simulink model "test4"  (R2021a)
settings: Solver=VariableStepAuto  StartTime=0.0  StopTime=20  RelTol=1e-1
undefined symbols (not defined in the file): B_EMB, C1, C_EMB, D_EMB, f, i_EMB, JL, JM, Jm_EMB, K1, N_EMB, rb_EMB, s_EMB, sigbuilder_block, Tc_EMB, Ts_EMB, ub_EMB
libraries: powerlib_extras x9, spsDCVoltageSourceLib x5, spsPermanentMagnetSynchronousMachineLib x5, spsUniversalBridgeLib x5, spspowerguiLib x5, spsVoltageMeasurementLib x4, pid_lib x4, simulink x3, dsparch4 x2, instrumentlib x2, Solver_SF x1
(part 2 of 3)

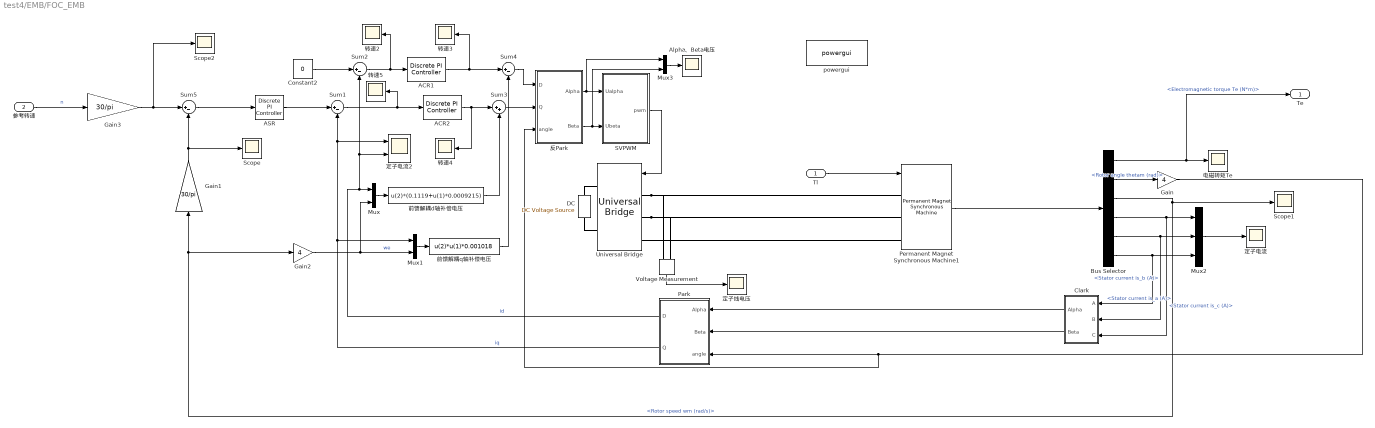
== system test4/EMB/FOC_EMB ==
  Tl : Inport
  参考转速 : Inport  Port=2
  ACR1 : powerlib_extras/Discrete  Control Blocks/Discrete PI Controller  Kp=4  Ki=80  Par_Limits=[560*0.9*sqrt(1/3) -560*0.9*sqrt(1/3)]  Init=0  Ts=1e-6
  ACR2 : powerlib_extras/Discrete  Control Blocks/Discrete PI Controller  Kp=4  Ki=80  Par_Limits=[560*0.9*sqrt(1/3) -560*0.9*sqrt(1/3)]  Init=0  Ts=1e-6
  ASR : powerlib_extras/Discrete  Control Blocks/Discrete PI Controller  Kp=5  Ki=200  Par_Limits=[65 -65]  Init=0  Ts=1e-6
  Alpha、Beta电压 : Scope
  Bus Selector : BusSelector  OutputSignals=Electromagnetic torque Te (N*m),Rotor angle thetam (rad),Rotor speed wm (rad/s),Stator current is_c (A),Stator current is_b (A),Stator current is_a (A)
  Clark : Subsystem
  Constant2 : Constant  Value=0
  DC : spsDCVoltageSourceLib/DC Voltage Source  Amplitude=560  Measurements=None
  Gain : Gain  Gain=4
  Gain1 : Gain  Gain=30/pi
  Gain2 : Gain  Gain=4
  Gain3 : Gain  Gain=30/pi
  Mux : Mux  Inputs=2
  Mux1 : Mux  Inputs=2
  Mux2 : Mux  Inputs=3
  Mux3 : Mux  Inputs=2
  Park : Subsystem
  Permanent Magnet Synchronous Machine1 : spsPermanentMagnetSynchronousMachineLib/Permanent Magnet Synchronous Machine  NbPhases=3  FluxDistribution=Sinusoidal  RotorType=Salient-pole  MechanicalLoad=Torque Tm  PresetModel=No  ShowDetailedParameters=on  MeasurementBus=off  Resistance=0.11  Inductance=8.5e-3  dqInductances=[0.0009215 0.001018]  La=0.000835  MachineConstant=Flux linkage established by magnets (V.s)  Flux=0.1119  VoltageCst=81.1857  TorqueCst=0.6714  Flat=120  Mechanical=[0.04 0.0002024 4 0]  PolePairs=4  InitialConditions=[0,0, 0,0]  InitialConditions5ph=[0 0 0 0 0 0]  RefAngle=Aligned with phase A axis (original Park)  IterativeDiscreteModel=Trapezoidal non iterative  TsBlock=-1  TsPowergui=0
  SVPWM : Subsystem
  Scope : Scope
  Scope1 : Scope
  Scope2 : Scope
  Sum{1..2,4..5} (4 alike) : Sum  Inputs=|+-
  Sum3 : Sum  Inputs=|++
  Universal Bridge : spsUniversalBridgeLib/Universal Bridge  Arms=3  SnubberResistance=1e5  SnubberCapacitance=inf  Device=IGBT / Diodes  Ron=1e-3  Lon=0  ForwardVoltages="[  0  0  ]"  ForwardVoltage=0  GTOparameters=[ 10e-6 , 20e-6 ]  IGBTparameters=[ 1e-6 , 2e-6 ]  Measurements=None  Measurements_2=None  converterType=Rectifier
  Voltage Measurement : spsVoltageMeasurementLib/Voltage Measurement  PhasorSimulation=off  OutputType=Complex  PSBequivalent=0
  powergui : spspowerguiLib/powergui  Priority=1  SimulationMode=Discrete  SampleTime=1e-6  frequency=60  Iterations=50  frequencyindice=0  Pbase=100e6  ErrMax=1e-4  UnitsV=kV  UnitsW=MW  buscounter=0  FunctionMessages=off  echomessages=off  EnableUseOfTLC=off  CurrentSourceSwitches=off  DisableSnubberDevices=off  DisableRonSwitches=off  DisableVfSwitches=off  DisplayEquations=off  AutomaticDiscreteSolvers=off  SolverType=Tustin  Interpol=off  ExternalGateDelay=off  methode=off  Ts=0  x0status=blocks  SPID=off  SwTol=0  HookPort=off  NonlinearTolerance=1e-4  nMaxIteration=100  ContinueOnMaxIteration=off  RestoreLinks=warning  ResistiveCurrentMeasurement=off  Frange=[0:2:500]  Ylog=off  Xlog=on  ShowGrid=off  save=off  variable=ZData  structure=ScopeData7  ZoomFFT=on  StartTime=2.5  cycles=3  DisplayStyle=1  fundamental=60  FreqAxis=off  MaxFrequency=2000  frequencyindicesteady=1  RmsSteady=1  display=off
  前馈解耦d轴补偿电压 : Fcn  Expr=u(2)*(0.1119+u(1)*0.0009215)
  前馈解耦q轴补偿电压 : Fcn  Expr=u(2)*u(1)*0.001018
  反Park : Subsystem
  定子电流 : Scope
  定子电流2 : Scope  NumInputPorts=2
  定子线电压 : Scope
  电磁转矩Te : Scope
  转速{2..5} (4 alike) : Scope
  Te : Outport
  wires:
  ACR1/1 -> 转速3/1, Sum4/1
  Bus Selector/4 -> Mux2/1, Clark/3(C)  "<Stator current is_c (A)>"
  Constant2/1 -> Sum2/1
  Gain/1 -> 反Park/3(angle), Park/3(angle)
  Gain2/1 -> Mux1/2, Mux/2  "we"
  Mux1/1 -> 前馈解耦q轴补偿电压/1
  SVPWM/1(pwm) -> Universal Bridge/1
  Sum4/1 -> 反Park/1(D)
  ACR2/1 -> 转速4/1, Sum3/1
  前馈解耦d轴补偿电压/1 -> Sum3/2
  参考转速/1 -> Gain3/1  "n"
  Bus Selector/2 -> Gain/1  "<Rotor angle thetam (rad)>"
  Bus Selector/5 -> Mux2/2, Clark/2(B)  "<Stator current is_b (A)>"
  Bus Selector/1 -> Te/1, 电磁转矩Te/1  "<Electromagnetic torque Te (N*m)>"
  Park/1(D) -> 定子电流2/2, Sum2/2, Mux/1  "id"
  Sum3/1 -> 反Park/2(Q)
  反Park/2(Beta) -> Mux3/2, SVPWM/2(Ubeta)
  Mux/1 -> 前馈解耦d轴补偿电压/1
  Bus Selector/3 -> Gain2/1, Gain1/1, Scope1/1  "<Rotor speed wm (rad/s)>"
  反Park/1(Alpha) -> Mux3/1, SVPWM/1(Ualpha)
  Mux3/1 -> Alpha、Beta电压/1
  Sum1/1 -> 转速5/1, ACR2/1
  Clark/2(Beta) -> Park/2(Beta)
  Park/2(Q) -> Mux1/1, 定子电流2/1, Sum1/2  "iq"
  Permanent Magnet Synchronous Machine1/1 -> Bus Selector/1
  Clark/1(Alpha) -> Park/1(Alpha)
  Sum5/1 -> ASR/1
  Bus Selector/6 -> Mux2/3, Clark/1(A)  "<Stator current is_a (A)>"
  Mux2/1 -> 定子电流/1
  Sum2/1 -> 转速2/1, ACR1/1
  前馈解耦q轴补偿电压/1 -> Sum4/2
  Voltage Measurement/1 -> 定子线电压/1
  Tl/1 -> Permanent Magnet Synchronous Machine1/1
  ASR/1 -> Sum1/1
  Gain1/1 -> Sum5/2, Scope/1
  Gain3/1 -> Scope2/1, Sum5/1
  connections:
  DC/LConn1 -- Universal Bridge/RConn2
  Permanent Magnet Synchronous Machine1/LConn3 -- Universal Bridge/LConn3
  DC/RConn1 -- Universal Bridge/RConn1
  Universal Bridge/LConn2 -- Permanent Magnet Synchronous Machine1/LConn2 -- Voltage Measurement/LConn2
  Universal Bridge/LConn1 -- Permanent Magnet Synchronous Machine1/LConn1 -- Voltage Measurement/LConn1

== system test4/EMB/Subsystem1 ==
  wm : Inport
  Fcl : Inport  Port=2
  TE : Inport  Port=3
  Constant : Constant  Value=D_EMB
  Constant1 : Constant  Value=C_EMB
  Constant2 : Constant  Value=Ts_EMB
  Constant3 : Constant  Value=Tc_EMB
  MATLAB Function : MATLAB Function  TreatAsAtomicUnit=on
  Tf : Outport
  wires:
  wm/1 -> MATLAB Function/1(wm)
  Fcl/1 -> MATLAB Function/2(Fcl)
  TE/1 -> MATLAB Function/3(TE)
  MATLAB Function/1(Tf) -> Tf/1
  Constant/1 -> MATLAB Function/4(D)
  Constant1/1 -> MATLAB Function/5(C)
  Constant2/1 -> MATLAB Function/6(Ts)
  Constant3/1 -> MATLAB Function/7(Tc)

== system test4/EMB/calculate_Fcl1 ==
  s : Inport
  MATLAB Function : MATLAB Function  TreatAsAtomicUnit=on
  Fcl : Outport
  wires:
  s/1 -> MATLAB Function/1(s)
  MATLAB Function/1(Fcl) -> Fcl/1

== system test4/EMB/行星齿轮+丝杆传动机构 ==
  Te : Inport
  TL1 : Inport  Port=2
  Tf : Inport  Port=3
  Add : Sum  Inputs=+---
  Add1 : Sum
  Constant : Constant  Value=B_EMB
  Gain : Gain  Gain=1/Jm_EMB
  Integrator : Integrator
  Product : Product
  dtheta : Outport
  Tl : Outport  Port=2
  wires:
  Te/1 -> Add/1
  TL1/1 -> Add1/1, Add/2
  Tf/1 -> Add1/2, Add/3
  Constant/1 -> Product/1
  Product/1 -> Add/4
  Gain/1 -> Integrator/1  "d2thetam"
  Add/1 -> Gain/1
  Integrator/1 -> dtheta/1, Product/2
  Add1/1 -> Tl/1

== system test4/EMB/计算丝杆位移 ==
  dtheta : Inport
  Constant : Constant  Value=s_EMB
  Constant1 : Constant  Value=i_EMB
  Divide : Product  Inputs=**/
  Gain : Gain  Gain=2*pi
  Integrator : Integrator
  s : Outport
  wires:
  dtheta/1 -> Divide/1
  Divide/1 -> Integrator/1  "ds/dt"
  Integrator/1 -> s/1
  Constant/1 -> Divide/2
  Gain/1 -> Divide/3
  Constant1/1 -> Gain/1

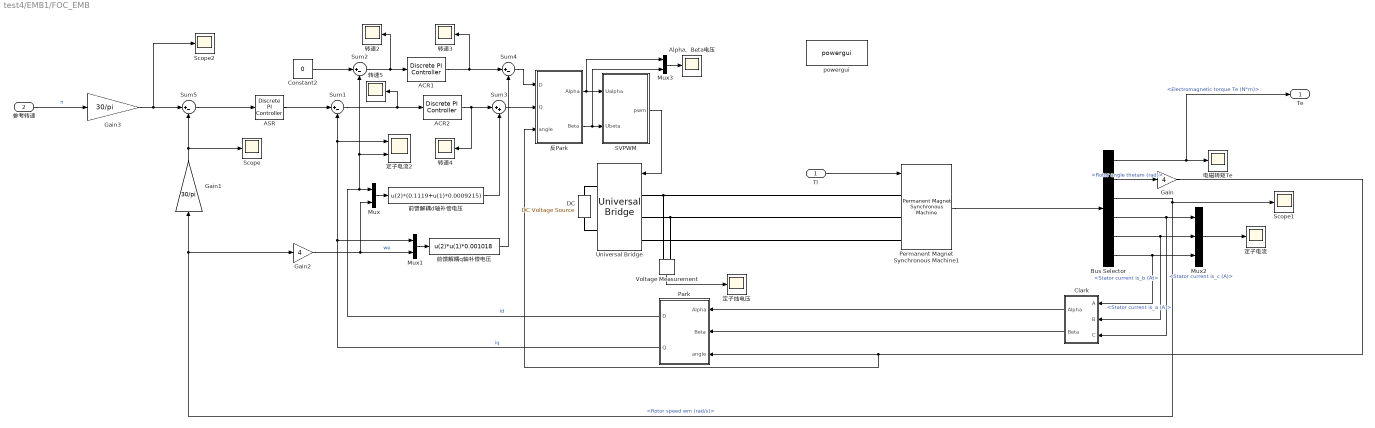
== system test4/EMB1/FOC_EMB ==
  Tl : Inport
  参考转速 : Inport  Port=2
  ACR1 : powerlib_extras/Discrete  Control Blocks/Discrete PI Controller  Kp=4  Ki=80  Par_Limits=[560*0.9*sqrt(1/3) -560*0.9*sqrt(1/3)]  Init=0  Ts=1e-6
  ACR2 : powerlib_extras/Discrete  Control Blocks/Discrete PI Controller  Kp=4  Ki=80  Par_Limits=[560*0.9*sqrt(1/3) -560*0.9*sqrt(1/3)]  Init=0  Ts=1e-6
  ASR : powerlib_extras/Discrete  Control Blocks/Discrete PI Controller  Kp=5  Ki=200  Par_Limits=[65 -65]  Init=0  Ts=1e-6
  Alpha、Beta电压 : Scope
  Bus Selector : BusSelector  OutputSignals=Electromagnetic torque Te (N*m),Rotor angle thetam (rad),Rotor speed wm (rad/s),Stator current is_c (A),Stator current is_b (A),Stator current is_a (A)
  Clark : Subsystem
  Constant2 : Constant  Value=0
  DC : spsDCVoltageSourceLib/DC Voltage Source  Amplitude=560  Measurements=None
  Gain : Gain  Gain=4
  Gain1 : Gain  Gain=30/pi
  Gain2 : Gain  Gain=4
  Gain3 : Gain  Gain=30/pi
  Mux : Mux  Inputs=2
  Mux1 : Mux  Inputs=2
  Mux2 : Mux  Inputs=3
  Mux3 : Mux  Inputs=2
  Park : Subsystem
  Permanent Magnet Synchronous Machine1 : spsPermanentMagnetSynchronousMachineLib/Permanent Magnet Synchronous Machine  NbPhases=3  FluxDistribution=Sinusoidal  RotorType=Salient-pole  MechanicalLoad=Torque Tm  PresetModel=No  ShowDetailedParameters=on  MeasurementBus=off  Resistance=0.11  Inductance=8.5e-3  dqInductances=[0.0009215 0.001018]  La=0.000835  MachineConstant=Flux linkage established by magnets (V.s)  Flux=0.1119  VoltageCst=81.1857  TorqueCst=0.6714  Flat=120  Mechanical=[0.04 0.0002024 4 0]  PolePairs=4  InitialConditions=[0,0, 0,0]  InitialConditions5ph=[0 0 0 0 0 0]  RefAngle=Aligned with phase A axis (original Park)  IterativeDiscreteModel=Trapezoidal non iterative  TsBlock=-1  TsPowergui=0
  SVPWM : Subsystem
  Scope : Scope
  Scope1 : Scope
  Scope2 : Scope
  Sum{1..2,4..5} (4 alike) : Sum  Inputs=|+-
  Sum3 : Sum  Inputs=|++
  Universal Bridge : spsUniversalBridgeLib/Universal Bridge  Arms=3  SnubberResistance=1e5  SnubberCapacitance=inf  Device=IGBT / Diodes  Ron=1e-3  Lon=0  ForwardVoltages="[  0  0  ]"  ForwardVoltage=0  GTOparameters=[ 10e-6 , 20e-6 ]  IGBTparameters=[ 1e-6 , 2e-6 ]  Measurements=None  Measurements_2=None  converterType=Rectifier
  Voltage Measurement : spsVoltageMeasurementLib/Voltage Measurement  PhasorSimulation=off  OutputType=Complex  PSBequivalent=0
  powergui : spspowerguiLib/powergui  Priority=1  SimulationMode=Discrete  SampleTime=1e-6  frequency=60  Iterations=50  frequencyindice=0  Pbase=100e6  ErrMax=1e-4  UnitsV=kV  UnitsW=MW  buscounter=0  FunctionMessages=off  echomessages=off  EnableUseOfTLC=off  CurrentSourceSwitches=off  DisableSnubberDevices=off  DisableRonSwitches=off  DisableVfSwitches=off  DisplayEquations=off  AutomaticDiscreteSolvers=off  SolverType=Tustin  Interpol=off  ExternalGateDelay=off  methode=off  Ts=0  x0status=blocks  SPID=off  SwTol=0  HookPort=off  NonlinearTolerance=1e-4  nMaxIteration=100  ContinueOnMaxIteration=off  RestoreLinks=warning  ResistiveCurrentMeasurement=off  Frange=[0:2:500]  Ylog=off  Xlog=on  ShowGrid=off  save=off  variable=ZData  structure=ScopeData7  ZoomFFT=on  StartTime=2.5  cycles=3  DisplayStyle=1  fundamental=60  FreqAxis=off  MaxFrequency=2000  frequencyindicesteady=1  RmsSteady=1  display=off
  前馈解耦d轴补偿电压 : Fcn  Expr=u(2)*(0.1119+u(1)*0.0009215)
  前馈解耦q轴补偿电压 : Fcn  Expr=u(2)*u(1)*0.001018
  反Park : Subsystem
  定子电流 : Scope
  定子电流2 : Scope  NumInputPorts=2
  定子线电压 : Scope
  电磁转矩Te : Scope
  转速{2..5} (4 alike) : Scope
  Te : Outport
  wires:
  Gain3/1 -> Sum5/1, Scope2/1
  Gain1/1 -> Scope/1, Sum5/2
  ASR/1 -> Sum1/1
  Tl/1 -> Permanent Magnet Synchronous Machine1/1
  Voltage Measurement/1 -> 定子线电压/1
  前馈解耦q轴补偿电压/1 -> Sum4/2
  Sum2/1 -> ACR1/1, 转速2/1
  Mux2/1 -> 定子电流/1
  Bus Selector/6 -> Clark/1(A), Mux2/3  "<Stator current is_a (A)>"
  Sum5/1 -> ASR/1
  Clark/1(Alpha) -> Park/1(Alpha)
  Permanent Magnet Synchronous Machine1/1 -> Bus Selector/1
  Park/2(Q) -> Sum1/2, 定子电流2/1, Mux1/1  "iq"
  Clark/2(Beta) -> Park/2(Beta)
  Sum1/1 -> ACR2/1, 转速5/1
  Mux3/1 -> Alpha、Beta电压/1
  反Park/1(Alpha) -> SVPWM/1(Ualpha), Mux3/1
  Bus Selector/3 -> Scope1/1, Gain1/1, Gain2/1  "<Rotor speed wm (rad/s)>"
  Mux/1 -> 前馈解耦d轴补偿电压/1
  反Park/2(Beta) -> SVPWM/2(Ubeta), Mux3/2
  Sum3/1 -> 反Park/2(Q)
  Park/1(D) -> Mux/1, Sum2/2, 定子电流2/2  "id"
  Bus Selector/1 -> 电磁转矩Te/1, Te/1  "<Electromagnetic torque Te (N*m)>"
  Bus Selector/5 -> Clark/2(B), Mux2/2  "<Stator current is_b (A)>"
  Bus Selector/2 -> Gain/1  "<Rotor angle thetam (rad)>"
  参考转速/1 -> Gain3/1  "n"
  前馈解耦d轴补偿电压/1 -> Sum3/2
  ACR2/1 -> Sum3/1, 转速4/1
  Sum4/1 -> 反Park/1(D)
  SVPWM/1(pwm) -> Universal Bridge/1
  Mux1/1 -> 前馈解耦q轴补偿电压/1
  Gain2/1 -> Mux/2, Mux1/2  "we"
  Gain/1 -> Park/3(angle), 反Park/3(angle)
  Constant2/1 -> Sum2/1
  Bus Selector/4 -> Clark/3(C), Mux2/1  "<Stator current is_c (A)>"
  ACR1/1 -> Sum4/1, 转速3/1
  connections:
  Voltage Measurement/LConn1 -- Permanent Magnet Synchronous Machine1/LConn1 -- Universal Bridge/LConn1
  Voltage Measurement/LConn2 -- Permanent Magnet Synchronous Machine1/LConn2 -- Universal Bridge/LConn2
  DC/RConn1 -- Universal Bridge/RConn1
  Permanent Magnet Synchronous Machine1/LConn3 -- Universal Bridge/LConn3
  DC/LConn1 -- Universal Bridge/RConn2

== system test4/EMB1/Subsystem1 ==
  wm : Inport
  Fcl : Inport  Port=2
  TE : Inport  Port=3
  Constant : Constant  Value=D_EMB
  Constant1 : Constant  Value=C_EMB
  Constant2 : Constant  Value=Ts_EMB
  Constant3 : Constant  Value=Tc_EMB
  MATLAB Function : MATLAB Function  TreatAsAtomicUnit=on
  Tf : Outport
  wires:
  Constant3/1 -> MATLAB Function/7(Tc)
  Constant2/1 -> MATLAB Function/6(Ts)
  Constant1/1 -> MATLAB Function/5(C)
  Constant/1 -> MATLAB Function/4(D)
  MATLAB Function/1(Tf) -> Tf/1
  TE/1 -> MATLAB Function/3(TE)
  Fcl/1 -> MATLAB Function/2(Fcl)
  wm/1 -> MATLAB Function/1(wm)

== system test4/EMB1/calculate_Fcl1 ==
  s : Inport
  MATLAB Function : MATLAB Function  TreatAsAtomicUnit=on
  Fcl : Outport
  wires:
  MATLAB Function/1(Fcl) -> Fcl/1
  s/1 -> MATLAB Function/1(s)

== system test4/EMB1/行星齿轮+丝杆传动机构 ==
  Te : Inport
  TL1 : Inport  Port=2
  Tf : Inport  Port=3
  Add : Sum  Inputs=+---
  Add1 : Sum
  Constant : Constant  Value=B_EMB
  Gain : Gain  Gain=1/Jm_EMB
  Integrator : Integrator
  Product : Product
  dtheta : Outport
  Tl : Outport  Port=2
  wires:
  Add1/1 -> Tl/1
  Integrator/1 -> Product/2, dtheta/1
  Add/1 -> Gain/1
  Gain/1 -> Integrator/1  "d2thetam"
  Product/1 -> Add/4
  Constant/1 -> Product/1
  Tf/1 -> Add/3, Add1/2
  TL1/1 -> Add/2, Add1/1
  Te/1 -> Add/1

== system test4/EMB1/计算丝杆位移 ==
  dtheta : Inport
  Constant : Constant  Value=s_EMB
  Constant1 : Constant  Value=i_EMB
  Divide : Product  Inputs=**/
  Gain : Gain  Gain=2*pi
  Integrator : Integrator
  s : Outport
  wires:
  Constant1/1 -> Gain/1
  Gain/1 -> Divide/3
  Constant/1 -> Divide/2
  Integrator/1 -> s/1
  Divide/1 -> Integrator/1  "ds/dt"
  dtheta/1 -> Divide/1

== system test4/传动系统模型1/Fcn1 ==
  TM : Inport
  d2theta1 : Inport  Port=2
  Add : Sum  Inputs=+---
  Add1 : Sum  Inputs=+-
  Add2 : Sum  Inputs=+-
  Gain : Gain  Gain=1/JM
  Gain1 : Gain  Gain=C1
  Gain2 : Gain  Gain=K1
  Integrator{,1..3} (4 alike) : Integrator
  Product : Product
  Scope2 : Scope
  电机阻尼系数 : Constant  Value=0.0002024
  d2theta : Outport
  dtheta : Outport  Port=2
  wires:
  Integrator1/1 -> Add2/1  "theta"
  Integrator2/1 -> Integrator3/1, Add1/2  "dtheta1"
  Integrator/1 -> dtheta/1, Product/1, Add1/1, Integrator1/1  "dtheta"
  Add/1 -> Gain/1
  Gain/1 -> Scope2/1, Integrator/1, d2theta/1  "d2theta"
  Add1/1 -> Gain1/1
  d2theta1/1 -> Integrator2/1
  Gain2/1 -> Add/4
  Add2/1 -> Gain2/1
  Integrator3/1 -> Add2/2  "theta1"
  Gain1/1 -> Add/3
  电机阻尼系数/1 -> Product/2
  TM/1 -> Add/1
  Product/1 -> Add/2

== system test4/传动系统模型1/Fcn2 ==
  TL : Inport
  d2thata : Inport  Port=2
  Add : Sum  Inputs=-++
  Add1 : Sum  Inputs=-+
  Add2 : Sum  Inputs=-+
  Gain : Gain  Gain=1/JL
  Gain1 : Gain  Gain=C1
  Gain2 : Gain  Gain=K1
  Integrator{,1..3} (4 alike) : Integrator
  Scope1 : Scope
  Scope2 : Scope
  d2thetaL : Outport
  dthetaL : Outport  Port=2
  wires:
  Gain1/1 -> Add/2
  Integrator3/1 -> Add2/2  "theta"
  Add2/1 -> Gain2/1
  Gain2/1 -> Add/3
  Add1/1 -> Scope2/1, Gain1/1
  Gain/1 -> Integrator/1, d2thetaL/1  "d2theta1"
  Add/1 -> Gain/1
  Integrator/1 -> dthetaL/1, Add1/1, Integrator1/1  "dtheta1"
  Integrator2/1 -> Scope1/1, Add1/2, Integrator3/1  "dtheta"
  Integrator1/1 -> Add2/1  "theta1"
  TL/1 -> Add/1
  d2thata/1 -> Integrator2/1

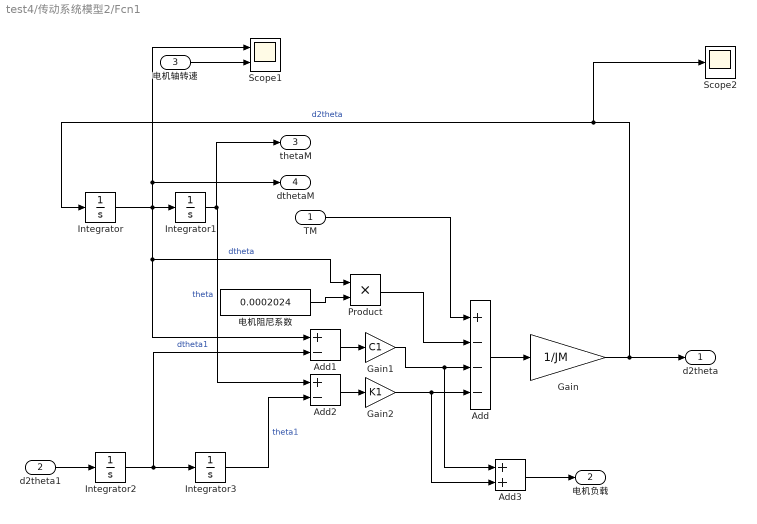
== system test4/传动系统模型2/Fcn1 ==
  TM : Inport
  d2theta1 : Inport  Port=2
  电机轴转速 : Inport  Port=3
  Add : Sum  Inputs=+---
  Add1 : Sum  Inputs=+-
  Add2 : Sum  Inputs=+-
  Add3 : Sum
  Gain : Gain  Gain=1/JM
  Gain1 : Gain  Gain=C1
  Gain2 : Gain  Gain=K1
  Integrator{,1..3} (4 alike) : Integrator
  Product : Product
  Scope1 : Scope  NumInputPorts=2
  Scope2 : Scope
  电机阻尼系数 : Constant  Value=0.0002024
  d2theta : Outport
  电机负载 : Outport  Port=2
  thetaM : Outport  Port=3
  dthetaM : Outport  Port=4
  wires:
  Add3/1 -> 电机负载/1
  Product/1 -> Add/2
  TM/1 -> Add/1
  电机阻尼系数/1 -> Product/2
  电机轴转速/1 -> Scope1/2
  Gain1/1 -> Add/3, Add3/1
  Integrator3/1 -> Add2/2  "theta1"
  Add2/1 -> Gain2/1
  Gain2/1 -> Add/4, Add3/2
  d2theta1/1 -> Integrator2/1
  Add1/1 -> Gain1/1
  Gain/1 -> d2theta/1, Integrator/1, Scope2/1  "d2theta"
  Add/1 -> Gain/1
  Integrator/1 -> Integrator1/1, Add1/1, Product/1, dthetaM/1, Scope1/1  "dtheta"
  Integrator2/1 -> Add1/2, Integrator3/1  "dtheta1"
  Integrator1/1 -> Add2/1, thetaM/1  "theta"

== system test4/传动系统模型2/Fcn2 ==
  TL : Inport
  d2thata : Inport  Port=2
  Add : Sum  Inputs=-++
  Add1 : Sum  Inputs=-+
  Add2 : Sum  Inputs=-+
  Gain : Gain  Gain=1/JL
  Gain1 : Gain  Gain=C1
  Gain2 : Gain  Gain=K1
  Integrator{,1..3} (4 alike) : Integrator
  Scope1 : Scope
  Scope2 : Scope
  d2thetaL : Outport
  thetaL : Outport  Port=2
  dthetaL : Outport  Port=3
  wires:
  d2thata/1 -> Integrator2/1
  TL/1 -> Add/1
  Integrator1/1 -> Add2/1, thetaL/1  "theta1"
  Integrator2/1 -> Integrator3/1, Add1/2, Scope1/1  "dtheta"
  Integrator/1 -> Integrator1/1, Add1/1, dthetaL/1  "dtheta1"
  Add/1 -> Gain/1
  Gain/1 -> d2thetaL/1, Integrator/1  "d2theta1"
  Add1/1 -> Gain1/1, Scope2/1
  Gain2/1 -> Add/3
  Add2/1 -> Gain2/1
  Integrator3/1 -> Add2/2  "theta"
  Gain1/1 -> Add/2

== system test4/传动系统模型2/轮胎模型 ==
  Input : Inport
  Output : Outport
  wires:
  Input/1 -> Output/1

== system test4/电机模型1/Clark ==
  A : Inport
  B : Inport  Port=2
  C : Inport  Port=3
  Add : Sum
  Add1 : Sum  Inputs=+-
  Add2 : Sum  Inputs=+-
  Gain : Gain  Gain=0.5
  Gain1 : Gain  Gain=2/3
  Gain2 : Gain  Gain=1/sqrt(3)
  Alpha : Outport
  Beta : Outport  Port=2
  wires:
  B/1 -> Add2/1, Add/1
  C/1 -> Add/2, Add2/2
  Add/1 -> Gain/1
  A/1 -> Add1/1
  Gain/1 -> Add1/2
  Add1/1 -> Gain1/1
  Gain1/1 -> Alpha/1
  Add2/1 -> Gain2/1
  Gain2/1 -> Beta/1

== system test4/电机模型1/Park ==
  Alpha : Inport
  Beta : Inport  Port=2
  angle : Inport  Port=3
  Add1 : Sum
  Add2 : Sum  Inputs=-+
  Product{,1..3} (4 alike) : Product
  Trigonometric Function1 : Trigonometry
  Trigonometric Function2 : Trigonometry  Operator=cos
  D : Outport
  Q : Outport  Port=2
  wires:
  Add2/1 -> Q/1
  Product3/1 -> Add2/2
  Product2/1 -> Add2/1
  Add1/1 -> D/1
  Product1/1 -> Add1/2
  Product/1 -> Add1/1
  Trigonometric Function1/1 -> Product2/2, Product1/2
  Beta/1 -> Product3/1, Product1/1
  Trigonometric Function2/1 -> Product3/2, Product/2
  Alpha/1 -> Product2/1, Product/1
  angle/1 -> Trigonometric Function1/1, Trigonometric Function2/1

== system test4/电机模型1/SVPWM ==
  Ualpha : Inport
  Ubeta : Inport  Port=2
  Constant : Constant  Value=0.0001
  Constant1 : Constant  Value=560
  PWM Generator : Subsystem
  Scope : Scope
  Scope1 : Scope
  Scope2 : Scope
  Sector Caculate : Subsystem
  T1T2 Caculate : Subsystem
  XYZ Caculate : Subsystem
  pwm : Outport
  wires:
  Ualpha/1 -> XYZ Caculate/1(Ualpha), Sector Caculate/1(Ualpha)
  Ubeta/1 -> Sector Caculate/2("Ubeta "), XYZ Caculate/2(Ubeta)
  Constant/1 -> PWM Generator/4(T3), T1T2 Caculate/3(Tpwm), XYZ Caculate/3(Ts)
  Constant1/1 -> XYZ Caculate/4(Udc)
  XYZ Caculate/1(XYZ) -> T1T2 Caculate/2(XYZ)
  Sector Caculate/1(N) -> Scope1/1, T1T2 Caculate/1(N), PWM Generator/1(N)
  T1T2 Caculate/1("T1 ") -> PWM Generator/2(T1), Scope2/1
  T1T2 Caculate/2(T2) -> PWM Generator/3(T2)
  PWM Generator/1(pwm) -> pwm/1, Scope/1

== system test4/电机模型1/反Park ==
  D : Inport
  Q : Inport  Port=2
  angle : Inport  Port=3
  Add1 : Sum  Inputs=+-
  Add2 : Sum
  Product{,1..3} (4 alike) : Product
  Trigonometric Function1 : Trigonometry
  Trigonometric Function2 : Trigonometry  Operator=cos
  Alpha : Outport
  Beta : Outport  Port=2
  wires:
  angle/1 -> Trigonometric Function2/1, Trigonometric Function1/1
  D/1 -> Product/1, Product2/1
  Trigonometric Function2/1 -> Product/2, Product3/2
  Q/1 -> Product1/1, Product3/1
  Trigonometric Function1/1 -> Product1/2, Product2/2
  Product/1 -> Add1/1
  Product1/1 -> Add1/2
  Add1/1 -> Alpha/1
  Product2/1 -> Add2/1
  Product3/1 -> Add2/2
  Add2/1 -> Beta/1

== system test4/路面负载转矩1/负载 ==
  Demux : Demux  Tag=STV Demux  Outputs=3
      settings: DisplayOption=none
  FromWs : FromWorkspace  Tag=STV FromWs  VariableName=tuvar
      SigBuilderData=|
      | common.afterFinalStr = 'Extrapolate'
      | common.sampleTime = 0
      | dataSet.timeRange = [0 10]
      | dataSet.name = 'Group 1'
      | sbobj.Groups.Name = 'Group 1'
      | sbobj.Groups.Signals(1).Name = 'Signal 1'
      | sbobj.Groups.Signals(1).XData = [0 0.1 0.1 10]
      | sbobj.Groups.Signals(1).YData = [0 0.1 20 20]
      | sbobj.Groups.Signals(2).Name = 'Signal 2'
      | sbobj.Groups.Signals(2).XData = [0 2 2 3 3 10]
      | sbobj.Groups.Signals(2).YData = [10 10 50 50 10 10]
      | sbobj.Groups.Signals(3).Name = 'Signal 3'
      | sbobj.Groups.Signals(3).XData = [0 10]
      | sbobj.Groups.Signals(3).YData = [10 10]
  Signal 1 : Outport  Tag=STV Outport
  Signal 2 : Outport  Tag=STV Outport  Port=2
  Signal 3 : Outport  Tag=STV Outport  Port=3
  wires:
  FromWs/1 -> Demux/1
  Demux/1 -> Signal 1/1
  Demux/2 -> Signal 2/1
  Demux/3 -> Signal 3/1

== system test4/驱动电机模型1/Clark ==
  A : Inport
  B : Inport  Port=2
  C : Inport  Port=3
  Add : Sum
  Add1 : Sum  Inputs=+-
  Add2 : Sum  Inputs=+-
  Gain : Gain  Gain=0.5
  Gain1 : Gain  Gain=2/3
  Gain2 : Gain  Gain=1/sqrt(3)
  Alpha : Outport
  Beta : Outport  Port=2
  wires:
  B/1 -> Add2/1, Add/1
  C/1 -> Add/2, Add2/2
  Add/1 -> Gain/1
  A/1 -> Add1/1
  Gain/1 -> Add1/2
  Add1/1 -> Gain1/1
  Gain1/1 -> Alpha/1
  Add2/1 -> Gain2/1
  Gain2/1 -> Beta/1

== system test4/驱动电机模型1/Park ==
  Alpha : Inport
  Beta : Inport  Port=2
  angle : Inport  Port=3
  Add1 : Sum
  Add2 : Sum  Inputs=-+
  Product{,1..3} (4 alike) : Product
  Trigonometric Function1 : Trigonometry
  Trigonometric Function2 : Trigonometry  Operator=cos
  D : Outport
  Q : Outport  Port=2
  wires:
  Add2/1 -> Q/1
  Product3/1 -> Add2/2
  Product2/1 -> Add2/1
  Add1/1 -> D/1
  Product1/1 -> Add1/2
  Product/1 -> Add1/1
  Trigonometric Function1/1 -> Product2/2, Product1/2
  Beta/1 -> Product3/1, Product1/1
  Trigonometric Function2/1 -> Product3/2, Product/2
  Alpha/1 -> Product2/1, Product/1
  angle/1 -> Trigonometric Function1/1, Trigonometric Function2/1

== system test4/驱动电机模型4/Clark ==
  A : Inport
  B : Inport  Port=2
  C : Inport  Port=3
  Add : Sum
  Add1 : Sum  Inputs=+-
  Add2 : Sum  Inputs=+-
  Gain : Gain  Gain=0.5
  Gain1 : Gain  Gain=2/3
  Gain2 : Gain  Gain=1/sqrt(3)
  Alpha : Outport
  Beta : Outport  Port=2
  wires:
  B/1 -> Add2/1, Add/1
  C/1 -> Add/2, Add2/2
  Add/1 -> Gain/1
  A/1 -> Add1/1
  Gain/1 -> Add1/2
  Add1/1 -> Gain1/1
  Gain1/1 -> Alpha/1
  Add2/1 -> Gain2/1
  Gain2/1 -> Beta/1

== system test4/驱动电机模型4/Park ==
  Alpha : Inport
  Beta : Inport  Port=2
  angle : Inport  Port=3
  Add1 : Sum
  Add2 : Sum  Inputs=-+
  Product{,1..3} (4 alike) : Product
  Trigonometric Function1 : Trigonometry
  Trigonometric Function2 : Trigonometry  Operator=cos
  D : Outport
  Q : Outport  Port=2
  wires:
  Add2/1 -> Q/1
  Product3/1 -> Add2/2
  Product2/1 -> Add2/1
  Add1/1 -> D/1
  Product1/1 -> Add1/2
  Product/1 -> Add1/1
  Trigonometric Function1/1 -> Product2/2, Product1/2
  Beta/1 -> Product3/1, Product1/1
  Trigonometric Function2/1 -> Product3/2, Product/2
  Alpha/1 -> Product2/1, Product/1
  angle/1 -> Trigonometric Function1/1, Trigonometric Function2/1

== system test4/EMB/FOC_EMB/Clark ==
  A : Inport
  B : Inport  Port=2
  C : Inport  Port=3
  Add : Sum
  Add1 : Sum  Inputs=+-
  Add2 : Sum  Inputs=+-
  Gain : Gain  Gain=0.5
  Gain1 : Gain  Gain=2/3
  Gain2 : Gain  Gain=1/sqrt(3)
  Alpha : Outport
  Beta : Outport  Port=2
  wires:
  B/1 -> Add2/1, Add/1
  C/1 -> Add/2, Add2/2
  Add/1 -> Gain/1
  A/1 -> Add1/1
  Gain/1 -> Add1/2
  Add1/1 -> Gain1/1
  Gain1/1 -> Alpha/1
  Add2/1 -> Gain2/1
  Gain2/1 -> Beta/1

== system test4/EMB/FOC_EMB/Park ==
  Alpha : Inport
  Beta : Inport  Port=2
  angle : Inport  Port=3
  Add1 : Sum
  Add2 : Sum  Inputs=-+
  Product{,1..3} (4 alike) : Product
  Trigonometric Function1 : Trigonometry
  Trigonometric Function2 : Trigonometry  Operator=cos
  D : Outport
  Q : Outport  Port=2
  wires:
  Add2/1 -> Q/1
  Product3/1 -> Add2/2
  Product2/1 -> Add2/1
  Add1/1 -> D/1
  Product1/1 -> Add1/2
  Product/1 -> Add1/1
  Trigonometric Function1/1 -> Product2/2, Product1/2
  Beta/1 -> Product3/1, Product1/1
  Trigonometric Function2/1 -> Product3/2, Product/2
  Alpha/1 -> Product2/1, Product/1
  angle/1 -> Trigonometric Function1/1, Trigonometric Function2/1

== system test4/EMB/FOC_EMB/SVPWM ==
  Ualpha : Inport
  Ubeta : Inport  Port=2
  Constant : Constant  Value=0.0001
  Constant1 : Constant  Value=560
  PWM Generator : Subsystem
  Scope : Scope
  Scope1 : Scope
  Scope2 : Scope
  Sector Caculate : Subsystem
  T1T2 Caculate : Subsystem
  XYZ Caculate : Subsystem
  pwm : Outport
  wires:
  Ualpha/1 -> XYZ Caculate/1(Ualpha), Sector Caculate/1(Ualpha)
  Ubeta/1 -> Sector Caculate/2("Ubeta "), XYZ Caculate/2(Ubeta)
  Constant/1 -> PWM Generator/4(T3), T1T2 Caculate/3(Tpwm), XYZ Caculate/3(Ts)
  Constant1/1 -> XYZ Caculate/4(Udc)
  XYZ Caculate/1(XYZ) -> T1T2 Caculate/2(XYZ)
  Sector Caculate/1(N) -> Scope1/1, T1T2 Caculate/1(N), PWM Generator/1(N)
  T1T2 Caculate/1("T1 ") -> PWM Generator/2(T1), Scope2/1
  T1T2 Caculate/2(T2) -> PWM Generator/3(T2)
  PWM Generator/1(pwm) -> pwm/1, Scope/1

== system test4/EMB/FOC_EMB/反Park ==
  D : Inport
  Q : Inport  Port=2
  angle : Inport  Port=3
  Add1 : Sum  Inputs=+-
  Add2 : Sum
  Product{,1..3} (4 alike) : Product
  Trigonometric Function1 : Trigonometry
  Trigonometric Function2 : Trigonometry  Operator=cos
  Alpha : Outport
  Beta : Outport  Port=2
  wires:
  angle/1 -> Trigonometric Function2/1, Trigonometric Function1/1
  D/1 -> Product/1, Product2/1
  Trigonometric Function2/1 -> Product/2, Product3/2
  Q/1 -> Product1/1, Product3/1
  Trigonometric Function1/1 -> Product1/2, Product2/2
  Product/1 -> Add1/1
  Product1/1 -> Add1/2
  Add1/1 -> Alpha/1
  Product2/1 -> Add2/1
  Product3/1 -> Add2/2
  Add2/1 -> Beta/1

== system test4/EMB1/FOC_EMB/Clark ==
  A : Inport
  B : Inport  Port=2
  C : Inport  Port=3
  Add : Sum
  Add1 : Sum  Inputs=+-
  Add2 : Sum  Inputs=+-
  Gain : Gain  Gain=0.5
  Gain1 : Gain  Gain=2/3
  Gain2 : Gain  Gain=1/sqrt(3)
  Alpha : Outport
  Beta : Outport  Port=2
  wires:
  Gain2/1 -> Beta/1
  Add2/1 -> Gain2/1
  Gain1/1 -> Alpha/1
  Add1/1 -> Gain1/1
  Gain/1 -> Add1/2
  A/1 -> Add1/1
  Add/1 -> Gain/1
  C/1 -> Add2/2, Add/2
  B/1 -> Add/1, Add2/1

== system test4/EMB1/FOC_EMB/Park ==
  Alpha : Inport
  Beta : Inport  Port=2
  angle : Inport  Port=3
  Add1 : Sum
  Add2 : Sum  Inputs=-+
  Product{,1..3} (4 alike) : Product
  Trigonometric Function1 : Trigonometry
  Trigonometric Function2 : Trigonometry  Operator=cos
  D : Outport
  Q : Outport  Port=2
  wires:
  angle/1 -> Trigonometric Function2/1, Trigonometric Function1/1
  Alpha/1 -> Product/1, Product2/1
  Trigonometric Function2/1 -> Product/2, Product3/2
  Beta/1 -> Product1/1, Product3/1
  Trigonometric Function1/1 -> Product1/2, Product2/2
  Product/1 -> Add1/1
  Product1/1 -> Add1/2
  Add1/1 -> D/1
  Product2/1 -> Add2/1
  Product3/1 -> Add2/2
  Add2/1 -> Q/1

== system test4/EMB1/FOC_EMB/SVPWM ==
  Ualpha : Inport
  Ubeta : Inport  Port=2
  Constant : Constant  Value=0.0001
  Constant1 : Constant  Value=560
  PWM Generator : Subsystem
  Scope : Scope
  Scope1 : Scope
  Scope2 : Scope
  Sector Caculate : Subsystem
  T1T2 Caculate : Subsystem
  XYZ Caculate : Subsystem
  pwm : Outport
  wires:
  PWM Generator/1(pwm) -> Scope/1, pwm/1
  T1T2 Caculate/2(T2) -> PWM Generator/3(T2)
  T1T2 Caculate/1("T1 ") -> Scope2/1, PWM Generator/2(T1)
  Sector Caculate/1(N) -> PWM Generator/1(N), T1T2 Caculate/1(N), Scope1/1
  XYZ Caculate/1(XYZ) -> T1T2 Caculate/2(XYZ)
  Constant1/1 -> XYZ Caculate/4(Udc)
  Constant/1 -> XYZ Caculate/3(Ts), T1T2 Caculate/3(Tpwm), PWM Generator/4(T3)
  Ubeta/1 -> XYZ Caculate/2(Ubeta), Sector Caculate/2("Ubeta ")
  Ualpha/1 -> Sector Caculate/1(Ualpha), XYZ Caculate/1(Ualpha)

== system test4/EMB1/FOC_EMB/反Park ==
  D : Inport
  Q : Inport  Port=2
  angle : Inport  Port=3
  Add1 : Sum  Inputs=+-
  Add2 : Sum
  Product{,1..3} (4 alike) : Product
  Trigonometric Function1 : Trigonometry
  Trigonometric Function2 : Trigonometry  Operator=cos
  Alpha : Outport
  Beta : Outport  Port=2
  wires:
  Add2/1 -> Beta/1
  Product3/1 -> Add2/2
  Product2/1 -> Add2/1
  Add1/1 -> Alpha/1
  Product1/1 -> Add1/2
  Product/1 -> Add1/1
  Trigonometric Function1/1 -> Product2/2, Product1/2
  Q/1 -> Product3/1, Product1/1
  Trigonometric Function2/1 -> Product3/2, Product/2
  D/1 -> Product2/1, Product/1
  angle/1 -> Trigonometric Function1/1, Trigonometric Function2/1

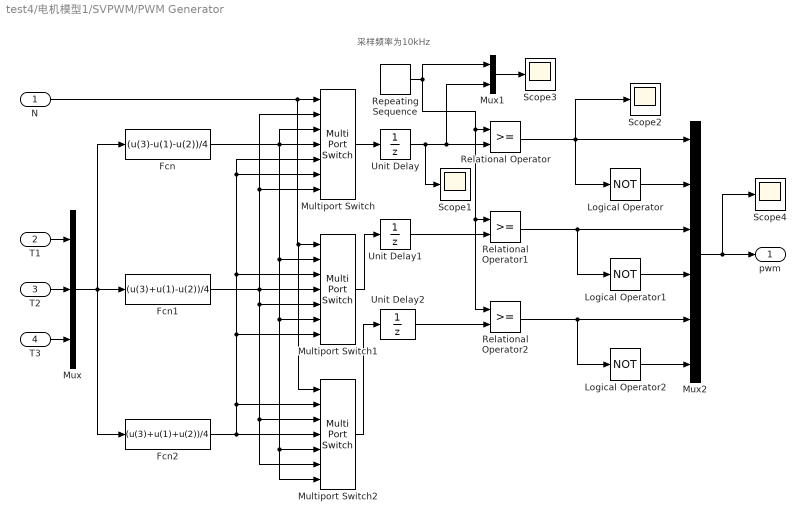
== system test4/电机模型1/SVPWM/PWM Generator ==
  note: 采样频率为10kHz
  N : Inport
  T1 : Inport  Port=2
  T2 : Inport  Port=3
  T3 : Inport  Port=4
  Fcn : Fcn  Expr=(u(3)-u(1)-u(2))/4
  Fcn1 : Fcn  Expr=(u(3)+u(1)-u(2))/4
  Fcn2 : Fcn  Expr=(u(3)+u(1)+u(2))/4
  Logical Operator : Logic  Operator=NOT  AllPortsSameDT=off  OutDataTypeStr=boolean
  Logical Operator1 : Logic  Operator=NOT  AllPortsSameDT=off  OutDataTypeStr=boolean
  Logical Operator2 : Logic  Operator=NOT  AllPortsSameDT=off  OutDataTypeStr=boolean
  Multiport Switch : MultiPortSwitch  Inputs=6  DiagnosticForDefault=None
  Multiport Switch1 : MultiPortSwitch  Inputs=6  DiagnosticForDefault=None
  Multiport Switch2 : MultiPortSwitch  Inputs=6  DiagnosticForDefault=None
  Mux : Mux  Inputs=3
  Mux1 : Mux  Inputs=2
  Mux2 : Mux  Inputs=6
  Relational Operator : RelationalOperator  OutDataTypeStr=boolean  RndMeth=Nearest
  Relational Operator1 : RelationalOperator  OutDataTypeStr=boolean  RndMeth=Nearest
  Relational Operator2 : RelationalOperator  OutDataTypeStr=boolean  RndMeth=Nearest
  Repeating Sequence : simulink/Sources/Repeating Sequence  rep_seq_t=[0 0.00005 0.0001]  rep_seq_y=[0 0.00005 0]
  Scope{1..4} (4 alike) : Scope
  Unit Delay : UnitDelay  SampleTime=0.0001  HasFrameUpgradeWarning=on
  Unit Delay1 : UnitDelay  SampleTime=0.0001  HasFrameUpgradeWarning=on
  Unit Delay2 : UnitDelay  SampleTime=0.0001  HasFrameUpgradeWarning=on
  pwm : Outport
  wires:
  T2/1 -> Mux/2
  T1/1 -> Mux/1
  T3/1 -> Mux/3
  Mux/1 -> Fcn/1, Fcn1/1, Fcn2/1
  N/1 -> Multiport Switch2/1, Multiport Switch1/1, Multiport Switch/1
  Fcn/1 -> Multiport Switch2/7, Multiport Switch2/5, Multiport Switch1/6, Multiport Switch1/2, Multiport Switch/4, Multiport Switch/3
  Fcn1/1 -> Multiport Switch/7, Multiport Switch/2, Multiport Switch2/6, Multiport Switch2/3, Multiport Switch1/5, Multiport Switch1/4
  Fcn2/1 -> Multiport Switch2/4, Multiport Switch2/2, Multiport Switch1/7, Multiport Switch1/3, Multiport Switch/6, Multiport Switch/5
  Repeating Sequence/1 -> Mux1/1, Relational Operator2/1, Relational Operator1/1, Relational Operator/1
  Relational Operator/1 -> Scope2/1, Logical Operator/1, Mux2/1
  Relational Operator1/1 -> Logical Operator1/1, Mux2/3
  Relational Operator2/1 -> Logical Operator2/1, Mux2/5
  Logical Operator/1 -> Mux2/2
  Logical Operator1/1 -> Mux2/4
  Logical Operator2/1 -> Mux2/6
  Mux2/1 -> Scope4/1, pwm/1
  Multiport Switch1/1 -> Unit Delay1/1
  Multiport Switch2/1 -> Unit Delay2/1
  Multiport Switch/1 -> Unit Delay/1
  Mux1/1 -> Scope3/1
  Unit Delay/1 -> Mux1/2, Relational Operator/2, Scope1/1
  Unit Delay1/1 -> Relational Operator1/2
  Unit Delay2/1 -> Relational Operator2/2

== system test4/电机模型1/SVPWM/Sector Caculate ==
  Ualpha : Inport
  "Ubeta " : Inport  Port=2
  Add : Sum  Inputs=+++
  Add1 : Sum  Inputs=+-
  Add2 : Sum  Inputs=--
  Constant : Constant
  Constant1 : Constant  Value=0
  Constant2 : Constant  Value=3/4
  Gain : Gain  Gain=4
  Gain1 : Gain  Gain=2
  Gain2 : Gain  Gain=0.5
  Product : Product
  Sqrt : Sqrt  SaturateOnIntegerOverflow=on
  Switch : Switch  Criteria=u2 > Threshold
  Switch1 : Switch  Criteria=u2 > Threshold
  Switch2 : Switch  Criteria=u2 > Threshold
  N : Outport
  wires:
  Ualpha/1 -> Product/1
  "Ubeta "/1 -> Switch/2, Gain2/1
  Add1/1 -> Switch1/2
  Add2/1 -> Switch2/2
  Constant/1 -> Switch/1, Switch1/1, Switch2/1
  Constant1/1 -> Switch2/3, Switch1/3, Switch/3
  Add/1 -> N/1
  Gain1/1 -> Add/2
  Gain/1 -> Add/3
  Switch2/1 -> Gain/1
  Switch1/1 -> Gain1/1
  Switch/1 -> Add/1
  Constant2/1 -> Sqrt/1
  Sqrt/1 -> Product/2
  Product/1 -> Add2/1, Add1/1
  Gain2/1 -> Add1/2, Add2/2

== system test4/电机模型1/SVPWM/T1T2 Caculate ==
  N : Inport
  XYZ : Inport  Port=2
  Tpwm : Inport  Port=3
  Demux : Demux  Outputs=3
  Divide : Product  Inputs=*/
  Divide1 : Product  Inputs=/*
  Gain : Gain  Gain=-1
  Gain1 : Gain  Gain=-1
  Gain2 : Gain  Gain=-1
  Multiport Switch : MultiPortSwitch  Inputs=6  DiagnosticForDefault=None
  Multiport Switch1 : MultiPortSwitch  Inputs=6  DiagnosticForDefault=None
  Product : Product
  Product1 : Product
  Subtract : Sum
  Subtract1 : Sum  Inputs=-+
  Switch : Switch  Criteria=u2 > Threshold
  Switch1 : Switch  Criteria=u2 > Threshold
  "T1 " : Outport
  T2 : Outport  Port=2
  wires:
  N/1 -> Multiport Switch1/1, Multiport Switch/1
  Demux/1 -> Multiport Switch1/4, Multiport Switch/6, Gain/1
  Demux/2 -> Multiport Switch/3, Multiport Switch1/2, Gain1/1
  Demux/3 -> Gain2/1, Multiport Switch1/5, Multiport Switch/2
  Gain/1 -> Multiport Switch/5, Multiport Switch1/3
  Gain1/1 -> Multiport Switch1/6, Multiport Switch/7
  Gain2/1 -> Multiport Switch1/7, Multiport Switch/4
  XYZ/1 -> Demux/1
  Multiport Switch/1 -> Switch/1, Product/1, Subtract/1  "T1"
  Multiport Switch1/1 -> Subtract/2, Product1/1, Switch1/1  "T2"
  Tpwm/1 -> Subtract1/2, Product/2, Product1/2
  Divide/1 -> Switch/3
  Divide1/1 -> Switch1/3
  Subtract1/1 -> Switch1/2, Switch/2
  Switch1/1 -> T2/1
  Switch/1 -> "T1 "/1
  Product/1 -> Divide/1
  Subtract/1 -> Divide/2, Divide1/1, Subtract1/1
  Product1/1 -> Divide1/2

== system test4/电机模型1/SVPWM/XYZ Caculate ==
  Ualpha : Inport
  Ubeta : Inport  Port=2
  Ts : Inport  Port=3
  Udc : Inport  Port=4
  Add : Sum
  Add1 : Sum  Inputs=+-
  Gain : Gain  Gain=3/2
  Gain1 : Gain  Gain=sqrt(3)
  Gain2 : Gain  Gain=sqrt(3)/2
  Math Function : Math  Operator=reciprocal  SignedPower=on  SaturateOnIntegerOverflow=on
  Mux : Mux  Inputs=3
  Product{,1..3} (4 alike) : Product
  XYZ : Outport
  wires:
  Ualpha/1 -> Gain/1
  Ubeta/1 -> Gain2/1, Gain1/1
  Ts/1 -> Product/1
  Udc/1 -> Math Function/1
  Math Function/1 -> Product/2
  Gain1/1 -> Product1/1
  Product1/1 -> Mux/1
  Product/1 -> Product1/2, Product2/2, Product3/2
  Product3/1 -> Mux/3
  Gain/1 -> Add/2, Add1/2
  Gain2/1 -> Add1/1, Add/1
  Add/1 -> Product2/1
  Add1/1 -> Product3/1
  Product2/1 -> Mux/2
  Mux/1 -> XYZ/1

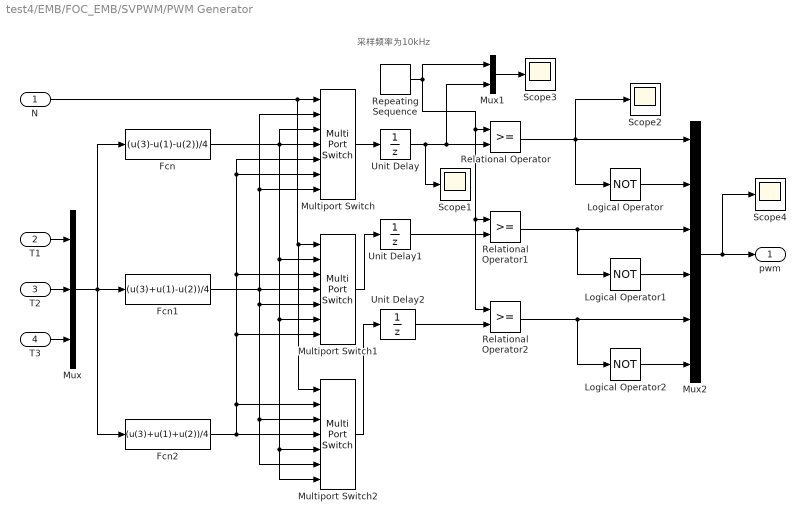
== system test4/EMB/FOC_EMB/SVPWM/PWM Generator ==
  note: 采样频率为10kHz
  N : Inport
  T1 : Inport  Port=2
  T2 : Inport  Port=3
  T3 : Inport  Port=4
  Fcn : Fcn  Expr=(u(3)-u(1)-u(2))/4
  Fcn1 : Fcn  Expr=(u(3)+u(1)-u(2))/4
  Fcn2 : Fcn  Expr=(u(3)+u(1)+u(2))/4
  Logical Operator : Logic  Operator=NOT  AllPortsSameDT=off  OutDataTypeStr=boolean
  Logical Operator1 : Logic  Operator=NOT  AllPortsSameDT=off  OutDataTypeStr=boolean
  Logical Operator2 : Logic  Operator=NOT  AllPortsSameDT=off  OutDataTypeStr=boolean
  Multiport Switch : MultiPortSwitch  Inputs=6  DiagnosticForDefault=None
  Multiport Switch1 : MultiPortSwitch  Inputs=6  DiagnosticForDefault=None
  Multiport Switch2 : MultiPortSwitch  Inputs=6  DiagnosticForDefault=None
  Mux : Mux  Inputs=3
  Mux1 : Mux  Inputs=2
  Mux2 : Mux  Inputs=6
  Relational Operator : RelationalOperator  OutDataTypeStr=boolean  RndMeth=Nearest
  Relational Operator1 : RelationalOperator  OutDataTypeStr=boolean  RndMeth=Nearest
  Relational Operator2 : RelationalOperator  OutDataTypeStr=boolean  RndMeth=Nearest
  Repeating Sequence : simulink/Sources/Repeating Sequence  rep_seq_t=[0 0.00005 0.0001]  rep_seq_y=[0 0.00005 0]
  Scope{1..4} (4 alike) : Scope
  Unit Delay : UnitDelay  SampleTime=0.0001  HasFrameUpgradeWarning=on
  Unit Delay1 : UnitDelay  SampleTime=0.0001  HasFrameUpgradeWarning=on
  Unit Delay2 : UnitDelay  SampleTime=0.0001  HasFrameUpgradeWarning=on
  pwm : Outport
  wires:
  T2/1 -> Mux/2
  T1/1 -> Mux/1
  T3/1 -> Mux/3
  Mux/1 -> Fcn/1, Fcn1/1, Fcn2/1
  N/1 -> Multiport Switch2/1, Multiport Switch1/1, Multiport Switch/1
  Fcn/1 -> Multiport Switch2/7, Multiport Switch2/5, Multiport Switch1/6, Multiport Switch1/2, Multiport Switch/4, Multiport Switch/3
  Fcn1/1 -> Multiport Switch/7, Multiport Switch/2, Multiport Switch2/6, Multiport Switch2/3, Multiport Switch1/5, Multiport Switch1/4
  Fcn2/1 -> Multiport Switch2/4, Multiport Switch2/2, Multiport Switch1/7, Multiport Switch1/3, Multiport Switch/6, Multiport Switch/5
  Repeating Sequence/1 -> Mux1/1, Relational Operator2/1, Relational Operator1/1, Relational Operator/1
  Relational Operator/1 -> Scope2/1, Logical Operator/1, Mux2/1
  Relational Operator1/1 -> Logical Operator1/1, Mux2/3
  Relational Operator2/1 -> Logical Operator2/1, Mux2/5
  Logical Operator/1 -> Mux2/2
  Logical Operator1/1 -> Mux2/4
  Logical Operator2/1 -> Mux2/6
  Mux2/1 -> Scope4/1, pwm/1
  Multiport Switch1/1 -> Unit Delay1/1
  Multiport Switch2/1 -> Unit Delay2/1
  Multiport Switch/1 -> Unit Delay/1
  Mux1/1 -> Scope3/1
  Unit Delay/1 -> Mux1/2, Relational Operator/2, Scope1/1
  Unit Delay1/1 -> Relational Operator1/2
  Unit Delay2/1 -> Relational Operator2/2

== system test4/EMB/FOC_EMB/SVPWM/Sector Caculate ==
  Ualpha : Inport
  "Ubeta " : Inport  Port=2
  Add : Sum  Inputs=+++
  Add1 : Sum  Inputs=+-
  Add2 : Sum  Inputs=--
  Constant : Constant
  Constant1 : Constant  Value=0
  Constant2 : Constant  Value=3/4
  Gain : Gain  Gain=4
  Gain1 : Gain  Gain=2
  Gain2 : Gain  Gain=0.5
  Product : Product
  Sqrt : Sqrt  SaturateOnIntegerOverflow=on
  Switch : Switch  Criteria=u2 > Threshold
  Switch1 : Switch  Criteria=u2 > Threshold
  Switch2 : Switch  Criteria=u2 > Threshold
  N : Outport
  wires:
  Ualpha/1 -> Product/1
  "Ubeta "/1 -> Switch/2, Gain2/1
  Add1/1 -> Switch1/2
  Add2/1 -> Switch2/2
  Constant/1 -> Switch/1, Switch1/1, Switch2/1
  Constant1/1 -> Switch2/3, Switch1/3, Switch/3
  Add/1 -> N/1
  Gain1/1 -> Add/2
  Gain/1 -> Add/3
  Switch2/1 -> Gain/1
  Switch1/1 -> Gain1/1
  Switch/1 -> Add/1
  Constant2/1 -> Sqrt/1
  Sqrt/1 -> Product/2
  Product/1 -> Add2/1, Add1/1
  Gain2/1 -> Add1/2, Add2/2

== system test4/EMB/FOC_EMB/SVPWM/T1T2 Caculate ==
  N : Inport
  XYZ : Inport  Port=2
  Tpwm : Inport  Port=3
  Demux : Demux  Outputs=3
  Divide : Product  Inputs=*/
  Divide1 : Product  Inputs=/*
  Gain : Gain  Gain=-1
  Gain1 : Gain  Gain=-1
  Gain2 : Gain  Gain=-1
  Multiport Switch : MultiPortSwitch  Inputs=6  DiagnosticForDefault=None
  Multiport Switch1 : MultiPortSwitch  Inputs=6  DiagnosticForDefault=None
  Product : Product
  Product1 : Product
  Subtract : Sum
  Subtract1 : Sum  Inputs=-+
  Switch : Switch  Criteria=u2 > Threshold
  Switch1 : Switch  Criteria=u2 > Threshold
  "T1 " : Outport
  T2 : Outport  Port=2
  wires:
  N/1 -> Multiport Switch1/1, Multiport Switch/1
  Demux/1 -> Multiport Switch1/4, Multiport Switch/6, Gain/1
  Demux/2 -> Multiport Switch/3, Multiport Switch1/2, Gain1/1
  Demux/3 -> Gain2/1, Multiport Switch1/5, Multiport Switch/2
  Gain/1 -> Multiport Switch/5, Multiport Switch1/3
  Gain1/1 -> Multiport Switch1/6, Multiport Switch/7
  Gain2/1 -> Multiport Switch1/7, Multiport Switch/4
  XYZ/1 -> Demux/1
  Multiport Switch/1 -> Switch/1, Product/1, Subtract/1  "T1"
  Multiport Switch1/1 -> Subtract/2, Product1/1, Switch1/1  "T2"
  Tpwm/1 -> Subtract1/2, Product/2, Product1/2
  Divide/1 -> Switch/3
  Divide1/1 -> Switch1/3
  Subtract1/1 -> Switch1/2, Switch/2
  Switch1/1 -> T2/1
  Switch/1 -> "T1 "/1
  Product/1 -> Divide/1
  Subtract/1 -> Divide/2, Divide1/1, Subtract1/1
  Product1/1 -> Divide1/2

== system test4/EMB/FOC_EMB/SVPWM/XYZ Caculate ==
  Ualpha : Inport
  Ubeta : Inport  Port=2
  Ts : Inport  Port=3
  Udc : Inport  Port=4
  Add : Sum
  Add1 : Sum  Inputs=+-
  Gain : Gain  Gain=3/2
  Gain1 : Gain  Gain=sqrt(3)
  Gain2 : Gain  Gain=sqrt(3)/2
  Math Function : Math  Operator=reciprocal  SignedPower=on  SaturateOnIntegerOverflow=on
  Mux : Mux  Inputs=3
  Product{,1..3} (4 alike) : Product
  XYZ : Outport
  wires:
  Ualpha/1 -> Gain/1
  Ubeta/1 -> Gain2/1, Gain1/1
  Ts/1 -> Product/1
  Udc/1 -> Math Function/1
  Math Function/1 -> Product/2
  Gain1/1 -> Product1/1
  Product1/1 -> Mux/1
  Product/1 -> Product1/2, Product2/2, Product3/2
  Product3/1 -> Mux/3
  Gain/1 -> Add/2, Add1/2
  Gain2/1 -> Add1/1, Add/1
  Add/1 -> Product2/1
  Add1/1 -> Product3/1
  Product2/1 -> Mux/2
  Mux/1 -> XYZ/1

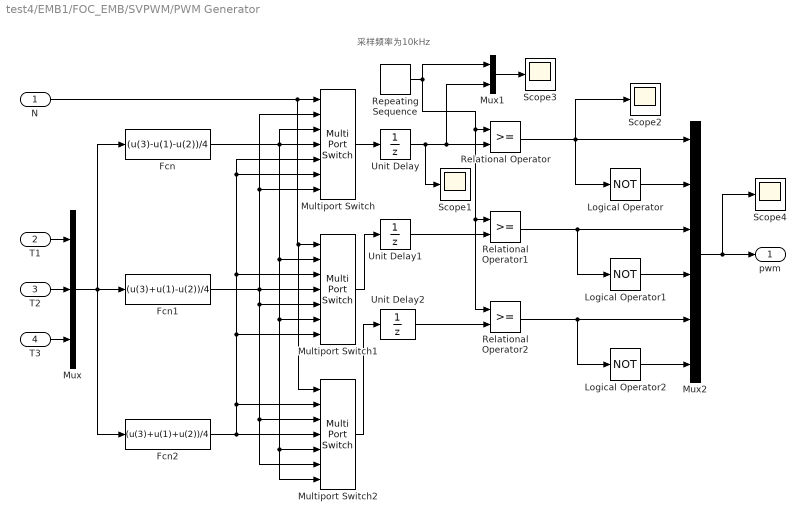
== system test4/EMB1/FOC_EMB/SVPWM/PWM Generator ==
  note: 采样频率为10kHz
  N : Inport
  T1 : Inport  Port=2
  T2 : Inport  Port=3
  T3 : Inport  Port=4
  Fcn : Fcn  Expr=(u(3)-u(1)-u(2))/4
  Fcn1 : Fcn  Expr=(u(3)+u(1)-u(2))/4
  Fcn2 : Fcn  Expr=(u(3)+u(1)+u(2))/4
  Logical Operator : Logic  Operator=NOT  AllPortsSameDT=off  OutDataTypeStr=boolean
  Logical Operator1 : Logic  Operator=NOT  AllPortsSameDT=off  OutDataTypeStr=boolean
  Logical Operator2 : Logic  Operator=NOT  AllPortsSameDT=off  OutDataTypeStr=boolean
  Multiport Switch : MultiPortSwitch  Inputs=6  DiagnosticForDefault=None
  Multiport Switch1 : MultiPortSwitch  Inputs=6  DiagnosticForDefault=None
  Multiport Switch2 : MultiPortSwitch  Inputs=6  DiagnosticForDefault=None
  Mux : Mux  Inputs=3
  Mux1 : Mux  Inputs=2
  Mux2 : Mux  Inputs=6
  Relational Operator : RelationalOperator  OutDataTypeStr=boolean  RndMeth=Nearest
  Relational Operator1 : RelationalOperator  OutDataTypeStr=boolean  RndMeth=Nearest
  Relational Operator2 : RelationalOperator  OutDataTypeStr=boolean  RndMeth=Nearest
  Repeating Sequence : simulink/Sources/Repeating Sequence  rep_seq_t=[0 0.00005 0.0001]  rep_seq_y=[0 0.00005 0]
  Scope{1..4} (4 alike) : Scope
  Unit Delay : UnitDelay  SampleTime=0.0001  HasFrameUpgradeWarning=on
  Unit Delay1 : UnitDelay  SampleTime=0.0001  HasFrameUpgradeWarning=on
  Unit Delay2 : UnitDelay  SampleTime=0.0001  HasFrameUpgradeWarning=on
  pwm : Outport
  wires:
  Unit Delay2/1 -> Relational Operator2/2
  Unit Delay1/1 -> Relational Operator1/2
  Unit Delay/1 -> Scope1/1, Relational Operator/2, Mux1/2
  Mux1/1 -> Scope3/1
  Multiport Switch/1 -> Unit Delay/1
  Multiport Switch2/1 -> Unit Delay2/1
  Multiport Switch1/1 -> Unit Delay1/1
  Mux2/1 -> pwm/1, Scope4/1
  Logical Operator2/1 -> Mux2/6
  Logical Operator1/1 -> Mux2/4
  Logical Operator/1 -> Mux2/2
  Relational Operator2/1 -> Mux2/5, Logical Operator2/1
  Relational Operator1/1 -> Mux2/3, Logical Operator1/1
  Relational Operator/1 -> Mux2/1, Logical Operator/1, Scope2/1
  Repeating Sequence/1 -> Relational Operator/1, Relational Operator1/1, Relational Operator2/1, Mux1/1
  Fcn2/1 -> Multiport Switch/5, Multiport Switch/6, Multiport Switch1/3, Multiport Switch1/7, Multiport Switch2/2, Multiport Switch2/4
  Fcn1/1 -> Multiport Switch1/4, Multiport Switch1/5, Multiport Switch2/3, Multiport Switch2/6, Multiport Switch/2, Multiport Switch/7
  Fcn/1 -> Multiport Switch/3, Multiport Switch/4, Multiport Switch1/2, Multiport Switch1/6, Multiport Switch2/5, Multiport Switch2/7
  N/1 -> Multiport Switch/1, Multiport Switch1/1, Multiport Switch2/1
  Mux/1 -> Fcn2/1, Fcn1/1, Fcn/1
  T3/1 -> Mux/3
  T1/1 -> Mux/1
  T2/1 -> Mux/2

== system test4/EMB1/FOC_EMB/SVPWM/Sector Caculate ==
  Ualpha : Inport
  "Ubeta " : Inport  Port=2
  Add : Sum  Inputs=+++
  Add1 : Sum  Inputs=+-
  Add2 : Sum  Inputs=--
  Constant : Constant
  Constant1 : Constant  Value=0
  Constant2 : Constant  Value=3/4
  Gain : Gain  Gain=4
  Gain1 : Gain  Gain=2
  Gain2 : Gain  Gain=0.5
  Product : Product
  Sqrt : Sqrt  SaturateOnIntegerOverflow=on
  Switch : Switch  Criteria=u2 > Threshold
  Switch1 : Switch  Criteria=u2 > Threshold
  Switch2 : Switch  Criteria=u2 > Threshold
  N : Outport
  wires:
  Gain2/1 -> Add2/2, Add1/2
  Product/1 -> Add1/1, Add2/1
  Sqrt/1 -> Product/2
  Constant2/1 -> Sqrt/1
  Switch/1 -> Add/1
  Switch1/1 -> Gain1/1
  Switch2/1 -> Gain/1
  Gain/1 -> Add/3
  Gain1/1 -> Add/2
  Add/1 -> N/1
  Constant1/1 -> Switch/3, Switch1/3, Switch2/3
  Constant/1 -> Switch2/1, Switch1/1, Switch/1
  Add2/1 -> Switch2/2
  Add1/1 -> Switch1/2
  "Ubeta "/1 -> Gain2/1, Switch/2
  Ualpha/1 -> Product/1

== system test4/EMB1/FOC_EMB/SVPWM/T1T2 Caculate ==
  N : Inport
  XYZ : Inport  Port=2
  Tpwm : Inport  Port=3
  Demux : Demux  Outputs=3
  Divide : Product  Inputs=*/
  Divide1 : Product  Inputs=/*
  Gain : Gain  Gain=-1
  Gain1 : Gain  Gain=-1
  Gain2 : Gain  Gain=-1
  Multiport Switch : MultiPortSwitch  Inputs=6  DiagnosticForDefault=None
  Multiport Switch1 : MultiPortSwitch  Inputs=6  DiagnosticForDefault=None
  Product : Product
  Product1 : Product
  Subtract : Sum
  Subtract1 : Sum  Inputs=-+
  Switch : Switch  Criteria=u2 > Threshold
  Switch1 : Switch  Criteria=u2 > Threshold
  "T1 " : Outport
  T2 : Outport  Port=2
  wires:
  Product1/1 -> Divide1/2
  Subtract/1 -> Subtract1/1, Divide1/1, Divide/2
  Product/1 -> Divide/1
  Switch/1 -> "T1 "/1
  Switch1/1 -> T2/1
  Subtract1/1 -> Switch/2, Switch1/2
  Divide1/1 -> Switch1/3
  Divide/1 -> Switch/3
  Tpwm/1 -> Product1/2, Product/2, Subtract1/2
  Multiport Switch1/1 -> Switch1/1, Product1/1, Subtract/2  "T2"
  Multiport Switch/1 -> Subtract/1, Product/1, Switch/1  "T1"
  XYZ/1 -> Demux/1
  Gain2/1 -> Multiport Switch/4, Multiport Switch1/7
  Gain1/1 -> Multiport Switch/7, Multiport Switch1/6
  Gain/1 -> Multiport Switch1/3, Multiport Switch/5
  Demux/3 -> Multiport Switch/2, Multiport Switch1/5, Gain2/1
  Demux/2 -> Gain1/1, Multiport Switch1/2, Multiport Switch/3
  Demux/1 -> Gain/1, Multiport Switch/6, Multiport Switch1/4
  N/1 -> Multiport Switch/1, Multiport Switch1/1

== system test4/EMB1/FOC_EMB/SVPWM/XYZ Caculate ==
  Ualpha : Inport
  Ubeta : Inport  Port=2
  Ts : Inport  Port=3
  Udc : Inport  Port=4
  Add : Sum
  Add1 : Sum  Inputs=+-
  Gain : Gain  Gain=3/2
  Gain1 : Gain  Gain=sqrt(3)
  Gain2 : Gain  Gain=sqrt(3)/2
  Math Function : Math  Operator=reciprocal  SignedPower=on  SaturateOnIntegerOverflow=on
  Mux : Mux  Inputs=3
  Product{,1..3} (4 alike) : Product
  XYZ : Outport
  wires:
  Mux/1 -> XYZ/1
  Product2/1 -> Mux/2
  Add1/1 -> Product3/1
  Add/1 -> Product2/1
  Gain2/1 -> Add/1, Add1/1
  Gain/1 -> Add1/2, Add/2
  Product3/1 -> Mux/3
  Product/1 -> Product3/2, Product2/2, Product1/2
  Product1/1 -> Mux/1
  Gain1/1 -> Product1/1
  Math Function/1 -> Product/2
  Udc/1 -> Math Function/1
  Ts/1 -> Product/1
  Ubeta/1 -> Gain1/1, Gain2/1
  Ualpha/1 -> Gain/1

== matlab function test4/EMB1/calculate_Fcl1/MATLAB Function ==
  data: s input; Fcl output
function Fcl = fcn(s)
s = s*1e3;  % 保留你的相对位移计算方式
Fcl =0;
% 按你的if-elseif顺序，补充s≤0的边界处理（避免Fcl未定义）
if s < 0.851 % 覆盖s≤0和0<s<0.851，均输出0（空行程/未触发）
    Fcl = 0;
elseif s >= 0.851 && s < 1.328  % 你的线性段条件
    Fcl = 312.603*s - 266.025;  % 保留你的乘法格式（标量适用）
elseif s >= 1.328 && s<=4  % 你的多项式段条件
    Fcl = -2017.2*s^3 + 16805*s^2 - 31759*s + 17412;  % 保留你的表达式
elseif s>4
    Fcl = 3.015520000000001e+04;
end

% 补充物理约束：确保夹紧力非负（符合实际制动逻辑，不破坏你的格式）
if Fcl < 0
    Fcl = 0;
end

end
